simulink model "PubIfDecisionVSM_HWA"  (R2020b)
settings: Solver=FixedStepAuto  StartTime=0.0  StopTime=Inf  RelTol=1e-3
PostLoadFcn:
  | if any(exist('dsrtsu_mdlpostloadfcn', 'file') ~= 0), dsrtsu_mdlpostloadfcn('Execute', bdroot); end
InitFcn:
  | , if any(exist('rtifpga_mdlclblib', 'file') ~= 0), rtifpga_mdlclblib('Init', bdroot); end,
  | , if any(exist('dsmpb_private', 'file') ~= 0), dsmpb_private('dsmpb_mdlclblib', 'Init', bdroot); end,
PreSaveFcn:
  | , if any(exist('dsmpb_private', 'file') ~= 0), dsmpb_private('dsmpb_mdlclblib', 'PreSave', bdroot); end,
CloseFcn:
  | , if any(exist('dsmpb_private', 'file') ~= 0), dsmpb_private('dsmpb_mdlclblib', 'Close', bdroot); end,
settings Model: DataDictionary=VSM_All.sldd  RTICANMMDATA=struct('GeneralSetupData',struct('modelroot','E:\HWA_Project\Git_ADAS_Store\Adas\VSM_Test\HWA','generalsettings',struct('filesettings',struct('destfolder',struct('Name','RTICANMM_FILES','Check',1),'buildfolder',struct('Name','.','Check',1),'AbsDestfolder',struct('Name','E:\HWA_Project\Git_ADAS_Store\Adas\VSM_Test\HWA\RTICANMM_FILES'),'AbsBuildfolder',struct('Name','E:\HWA_Project\Git_ADAS_Store\Adas\VSM_Test\HWA'))),'options',struct('addpaths',1,'rmpaths',1,'addtrcexclusion',false,'cannavigator',struct('checkmonitoring',0),'show_usrtrc',0,'use_usrtrc',0),'advanced',struct('options',ones(1,100)),'MPSetup',{{}},'RTI',struct('Type','DSRT','Ver','4.4','Date','02-Nov-2020'),'modelname','PubIfDecisionVSM_HWA','block','PubIfDecisionVSM_HWA'))  DSRTSU_INTERNAL_RTIFPGA=170  Creator=GW00180895  LastModifiedBy=GW00201299
settings OptimizationCC: BlockReduction=off  ConditionallyExecuteInputs=off  OptimizeBlockIOStorage=off  BufferReuse=off  GlobalBufferReuse=off  ExpressionFolding=off  LocalBlockOutputs=off  OptimizeDataStoreBuffers=off  BusAssignmentInplaceUpdate=off
settings DebuggingCC: TasksWithSamePriorityMsg=none
settings HardwareCC: ProdBitPerPointer=32  ProdBitPerSizeT=32  ProdBitPerPtrDiffT=32  ProdLargestAtomicInteger=Integer  ProdWordSize=32  ProdHWDeviceType=Custom Processor->Custom
settings ModelReferenceCC: UpdateModelReferenceTargets=IfOutOfDate  EnableParallelModelReferenceBuilds=on  ModelReferenceNumInstancesAllowed=Single
settings SFSimCC: MATLABDynamicMemAlloc=off
settings RTWCC: Description=dSPACE Run-Time Target (for VEOS on Windows and ConfigurationDesk)  SystemTargetFile=dsrt.tlc  GenCodeOnly=on  MakeCommand=make_dsrt  TemplateMakefile=dsrt_default_tmf  RTWVerbose=off
settings CodeAppCC: MaxIdLength=128
settings STFCustomTargetCC: TargetLangStandard=C99 (ISO)  ParMdlRefBuildCompliant=on  ConcurrentExecutionCompliant=off  CPPClassGenCompliant=off  GRTInterface=off  SystemTargetFile=dsrt.tlc
settings GRTTargetCC: CompOptLevelCompliant=off  ConcurrentExecutionCompliant=off  CombineOutputUpdateFcns=off  MatFileLogging=off  CPPClassGenCompliant=off  UseToolchainInfoCompliant=off

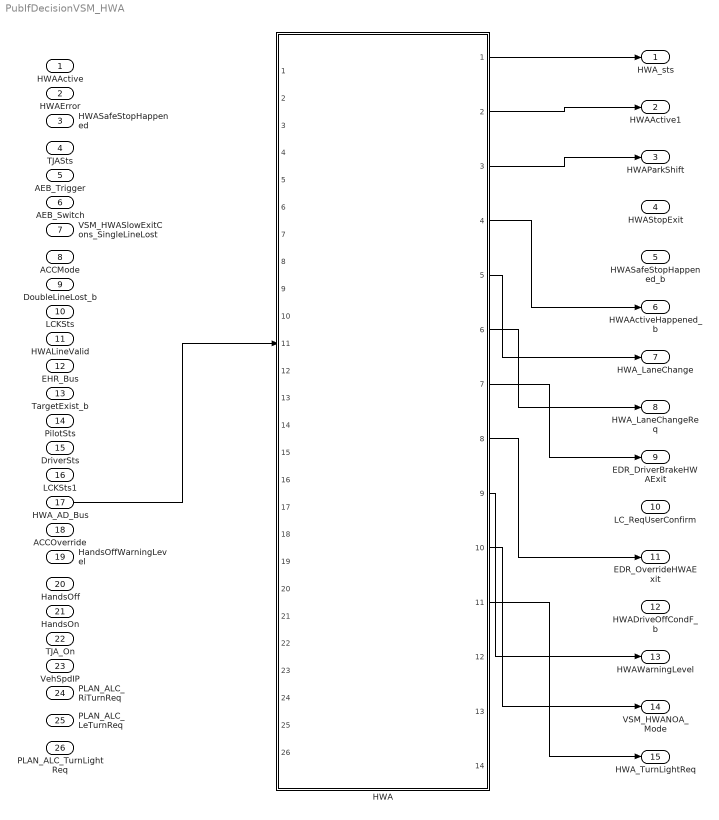
== system PubIfDecisionVSM_HWA ==
  HWAActive : Inport  OutDataTypeStr=boolean
  HWAError : Inport  Port=2  OutDataTypeStr=uint8
  HWASafeStopHappened : Inport  Port=3  OutDataTypeStr=boolean
  TJASts : Inport  Port=4  OutDataTypeStr=Enum: TJA_STATE
  AEB_Trigger : Inport  Port=5  OutDataTypeStr=boolean
  AEB_Switch : Inport  Port=6  OutDataTypeStr=boolean
  VSM_HWASlowExitCons_SingleLineLost : Inport  Port=7  OutDataTypeStr=boolean
  ACCMode : Inport  Port=8  OutDataTypeStr=Enum: ACC_STATE
  DoubleLineLost_b : Inport  Port=9  OutDataTypeStr=boolean
  LCKSts : Inport  Port=10  OutDataTypeStr=Enum: LCK_STATE
  HWALineValid : Inport  Port=11  OutDataTypeStr=boolean
  EHR_Bus : Inport  Port=12  OutDataTypeStr=Bus: EHR_Bus
  TargetExist_b : Inport  Port=13  OutDataTypeStr=boolean
  PilotSts : Inport  Port=14  OutDataTypeStr=uint8
  DriverSts : Inport  Port=15  OutDataTypeStr=uint8
  LCKSts1 : Inport  Port=16  OutDataTypeStr=Enum: LCK_STATE
  HWA_AD_Bus : Inport  Port=17  OutDataTypeStr=Bus: HWA_AD_Bus
  ACCOverride : Inport  Port=18  OutDataTypeStr=boolean
  HandsOffWarningLevel : Inport  Port=19  OutDataTypeStr=uint8
  HandsOff : Inport  Port=20  OutDataTypeStr=boolean
  HandsOn : Inport  Port=21  OutDataTypeStr=boolean
  TJA_On : Inport  Port=22  OutDataTypeStr=boolean
  VehSpdIP : Inport  Port=23  OutDataTypeStr=single
  PLAN_ALC_RiTurnReq : Inport  Port=24  OutDataTypeStr=uint8
  PLAN_ALC_LeTurnReq : Inport  Port=25  OutDataTypeStr=uint8
  PLAN_ALC_TurnLightReq : Inport  Port=26
  HWA : Subsystem  ReferencedSubsystem=PvtSubSys_VSM_HWA_DHT
  HWA_sts : Outport  OutDataTypeStr=Enum: HWA_STATE
  HWAActive1 : Outport  Port=2  OutDataTypeStr=boolean
  HWAParkShift : Outport  Port=3  OutDataTypeStr=boolean
  HWAStopExit : Outport  Port=4  OutDataTypeStr=boolean
  HWASafeStopHappened_b : Outport  Port=5  OutDataTypeStr=boolean
  HWAActiveHappened_b : Outport  Port=6  OutDataTypeStr=boolean
  HWA_LaneChange : Outport  Port=7  OutDataTypeStr=uint8
  HWA_LaneChangeReq : Outport  Port=8  OutDataTypeStr=uint8
  EDR_DriverBrakeHWAExit : Outport  Port=9  OutDataTypeStr=boolean
  LC_ReqUserConfirm : Outport  Port=10  OutDataTypeStr=boolean
  EDR_OverrideHWAExit : Outport  Port=11  OutDataTypeStr=boolean
  HWADriveOffCondF_b : Outport  Port=12  OutDataTypeStr=boolean
  HWAWarningLevel : Outport  Port=13  OutDataTypeStr=uint8
  VSM_HWANOA_Mode : Outport  Port=14  OutDataTypeStr=uint8
  HWA_TurnLightReq : Outport  Port=15
  wires:
  HWA/5 -> HWA_LaneChange/1
  HWA/4 -> HWAActiveHappened_b/1
  HWA/6 -> HWA_LaneChangeReq/1
  ? -> HWASafeStopHappened_b/1
  HWA/7 -> EDR_DriverBrakeHWAExit/1
  ? -> LC_ReqUserConfirm/1
  ? -> HWAStopExit/1
  HWA/3 -> HWAParkShift/1
  HWA/8 -> EDR_OverrideHWAExit/1
  HWA/2 -> HWAActive1/1
  ? -> HWADriveOffCondF_b/1
  HWA/1 -> HWA_sts/1
  HWA/9 -> HWAWarningLevel/1
  HWA/10 -> VSM_HWANOA_Mode/1
  HWA/11 -> HWA_TurnLightReq/1
  HWA_AD_Bus/1 -> HWA/11
